simulink model "Frank_feedback"  (Simulink 8.3)
settings: Solver=ode4  StartTime=0.0  StopTime=30  FixedStep=Ts  RelTol=1e-3
values from neighbouring files (symbols this model uses):
  Ts = 0.001    [init_frank.m]
undefined symbols (not defined in the file or in its folder): K_lqr, Kt, R, rob_str, W
undefined symbols (not defined in the file): prjname
(part 1 of 2)
settings Model: Creator=parallels  LastModifiedBy=parallels
settings DataIOCC: SignalLoggingSaveFormat=Dataset
settings DebuggingCC: UnderspecifiedInitializationDetection=Simplified  StateNameClashWarn=none
settings GRTTargetCC: CombineOutputUpdateFcns=on  GRTInterface=off

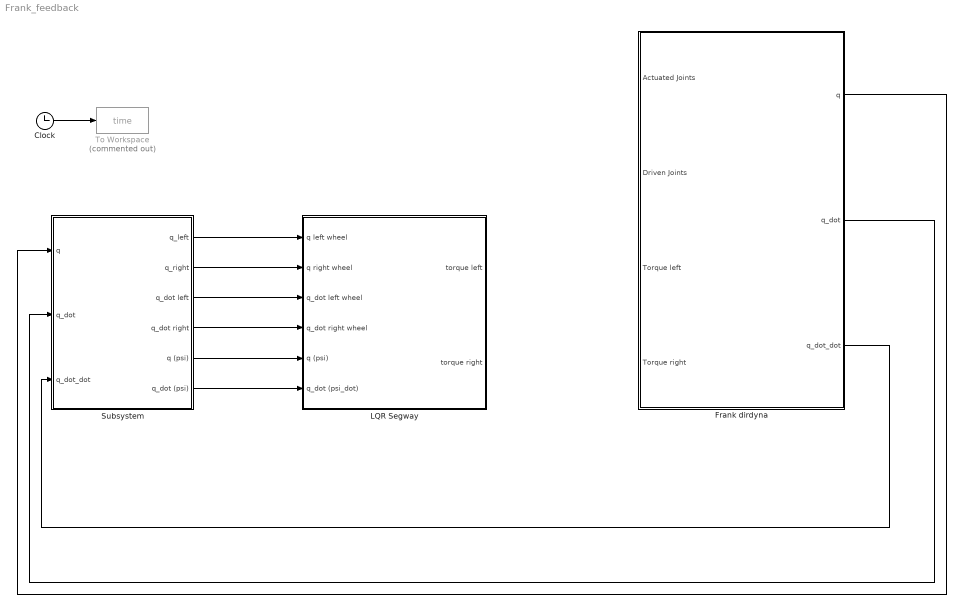
== system Frank_feedback ==
  Clock : Clock
  Frank dirdyna : Subsystem
  LQR Segway : Subsystem
  Subsystem : Subsystem
  To Workspace : ToWorkspace  Commented=on  VariableName=time  SampleTime=-1
  wires:
  Subsystem/1(q_left) -> LQR Segway/1("q left wheel ")
  Subsystem/2(q_right) -> LQR Segway/2(q right wheel)
  Subsystem/3(q_dot left) -> LQR Segway/3(q_dot left wheel)
  Subsystem/4(q_dot right) -> LQR Segway/4(q_dot right wheel)
  Subsystem/5(q (psi)) -> LQR Segway/5(q (psi))
  Subsystem/6(q_dot (psi)) -> LQR Segway/6("q_dot (psi_dot) ")
  Frank dirdyna/3(q_dot_dot) -> Subsystem/3(q_dot_dot)
  Frank dirdyna/2(q_dot) -> Subsystem/2(q_dot)
  Frank dirdyna/1(q) -> Subsystem/1(q)
  Clock/1 -> To Workspace/1

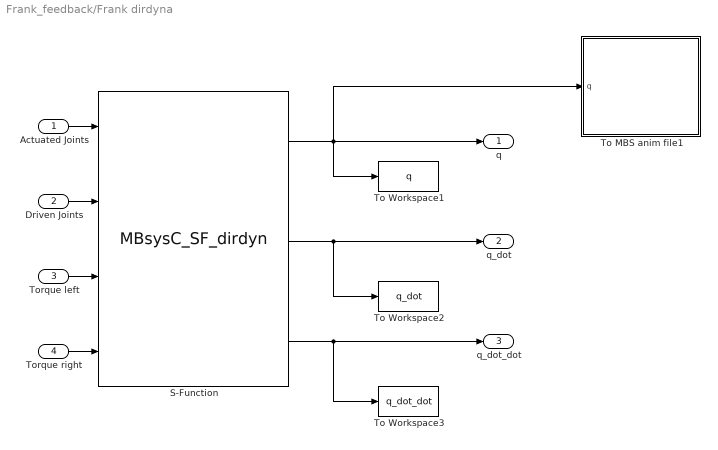
== system Frank_feedback/Frank dirdyna ==
  Actuated Joints : Inport
  Driven Joints : Inport  Port=2
  Torque left : Inport  Port=3
  Torque right : Inport  Port=4
  S-Function : S-Function  FunctionName=MBsysC_SF_dirdyn  Parameters='/home/parallels/Documents/MBProjects/Frank_segway/dataR/Frank_segway.mbs'  EnableBusSupport=off
  To MBS anim file1 : Subsystem  AncestorBlock=Robotran/Utilities/To MBS anim file  StopFcn=|  mask{varname=tqres, filename=simdir.anim, overwrite=0, samplingRate=1000, prjname=prjname}
      | varname = get_param(gcb,'varname');                                     
      | filename = get_param(gcb,'filename');                                   
      | tq = evalin('base',varname);                                            
      | tt = tq.time;                                                           
      | qq = tq.signals.values;                                                 
      | userData = get_param(gcb,'UserData');                                   
      | mbs_data = MBS_data;                                           
      | mbs_info = MBS_info;                                           
      | overwrite = str2double(get_param(gcb,'overwrite'));                     
      |                                                                         
      | samplingRate = str2double(get_param(gcb,'samplingRate'));               
      | mbs_gen_simdir(prjname,tt,qq,filename,overwrite,samplingRate);
      mask prompts: varname "variable name"; filename "anim file name"; overwrite "overwrite flag"; samplingRate "sampling rate"
      settings: CopyFcn=MBStoAnimFile_v2;  OpenFcn=MBStoAnimFile_v2;
      mask Display: image(imread('Logo_anim.jpg'))
  To Workspace1 : ToWorkspace  VariableName=q  SampleTime=-1
  To Workspace2 : ToWorkspace  VariableName=q_dot  SampleTime=-1
  To Workspace3 : ToWorkspace  VariableName=q_dot_dot  SampleTime=-1
  q : Outport
  q_dot : Outport  Port=2
  q_dot_dot : Outport  Port=3
  wires:
  Actuated Joints/1 -> S-Function/1
  Driven Joints/1 -> S-Function/2
  Torque left/1 -> S-Function/3
  Torque right/1 -> S-Function/4
  S-Function/1 -> To MBS anim file1/1(q), q/1, To Workspace1/1
  S-Function/2 -> To Workspace2/1, q_dot/1
  S-Function/3 -> q_dot_dot/1, To Workspace3/1

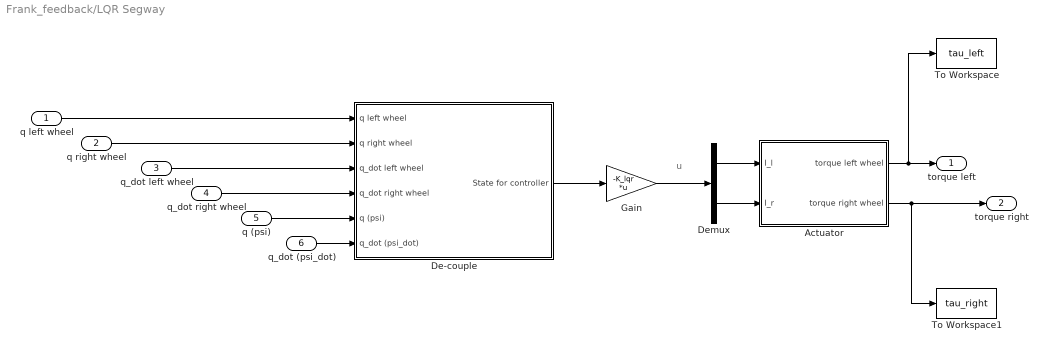
== system Frank_feedback/LQR Segway ==
  note: u
  "q left wheel " : Inport
  q right wheel : Inport  Port=2
  q_dot left wheel : Inport  Port=3
  q_dot right wheel : Inport  Port=4
  q (psi) : Inport  Port=5
  "q_dot (psi_dot) " : Inport  Port=6
  Actuator : Subsystem
  De-couple : Subsystem
  Demux : Demux  Outputs=2
  Gain : Gain  Gain=-K_lqr  Multiplication=Matrix(K*u) (u vector)
  To Workspace : ToWorkspace  VariableName=tau_left  SampleTime=-1
  To Workspace1 : ToWorkspace  VariableName=tau_right  SampleTime=-1
  torque left : Outport
  torque right : Outport  Port=2
  wires:
  "q left wheel "/1 -> De-couple/1("q left wheel ")
  q right wheel/1 -> De-couple/2(q right wheel)
  q_dot left wheel/1 -> De-couple/3(q_dot left wheel)
  q_dot right wheel/1 -> De-couple/4(q_dot right wheel)
  De-couple/1(State for controller) -> Gain/1
  q (psi)/1 -> De-couple/5(q (psi))
  "q_dot (psi_dot) "/1 -> De-couple/6("q_dot (psi_dot) ")
  Gain/1 -> Demux/1
  Actuator/1(torque left wheel) -> To Workspace/1, torque left/1
  Demux/1 -> Actuator/1(I_l)
  Demux/2 -> Actuator/2(I_r)
  Actuator/2(torque right wheel) -> To Workspace1/1, torque right/1

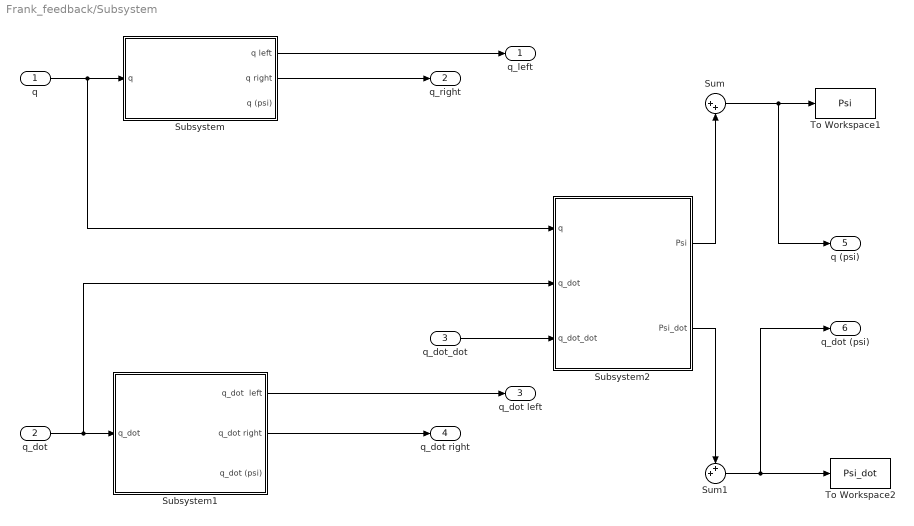
== system Frank_feedback/Subsystem ==
  q : Inport
  q_dot : Inport  Port=2
  q_dot_dot : Inport  Port=3
  Subsystem : Subsystem
  Subsystem1 : Subsystem
  Subsystem2 : Subsystem
  Sum : Sum  Inputs=|++
  Sum1 : Sum  Inputs=++|
  To Workspace1 : ToWorkspace  VariableName=Psi  SampleTime=-1
  To Workspace2 : ToWorkspace  VariableName=Psi_dot  SampleTime=-1
  q_left : Outport
  q_right : Outport  Port=2
  q_dot left : Outport  Port=3
  q_dot right : Outport  Port=4
  q (psi) : Outport  Port=5
  q_dot (psi) : Outport  Port=6
  wires:
  q/1 -> Subsystem2/1(q), Subsystem/1(q)
  Subsystem/2(q right) -> q_right/1
  Subsystem/1(q left) -> q_left/1
  q_dot/1 -> Subsystem2/2(q_dot), Subsystem1/1(q_dot)
  Subsystem1/2(q_dot right) -> q_dot right/1
  Subsystem1/1(q_dot  left) -> q_dot left/1
  q_dot_dot/1 -> Subsystem2/3(q_dot_dot)
  Sum1/1 -> q_dot (psi)/1, To Workspace2/1
  Sum/1 -> q (psi)/1, To Workspace1/1
  Subsystem2/1(Psi) -> Sum/2
  Subsystem2/2(Psi_dot) -> Sum1/1

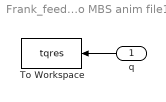
== system Frank_feedback/Frank dirdyna/To MBS anim file1 ==
  q : Inport
  To Workspace : ToWorkspace  VariableName=tqres  SaveFormat=Structure With Time  SampleTime=-1
  wires:
  q/1 -> To Workspace/1

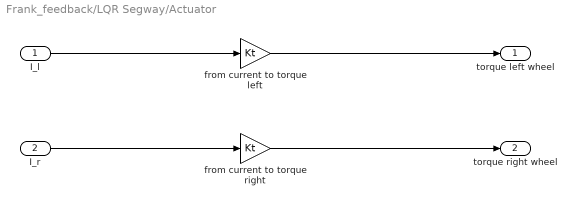
== system Frank_feedback/LQR Segway/Actuator ==
  I_l : Inport
  I_r : Inport  Port=2
  from current to torque left : Gain  Gain=Kt
  from current to torque right : Gain  Gain=Kt
  torque left wheel : Outport
  torque right wheel : Outport  Port=2
  wires:
  I_l/1 -> from current to torque left/1
  I_r/1 -> from current to torque right/1
  from current to torque left/1 -> torque left wheel/1
  from current to torque right/1 -> torque right wheel/1

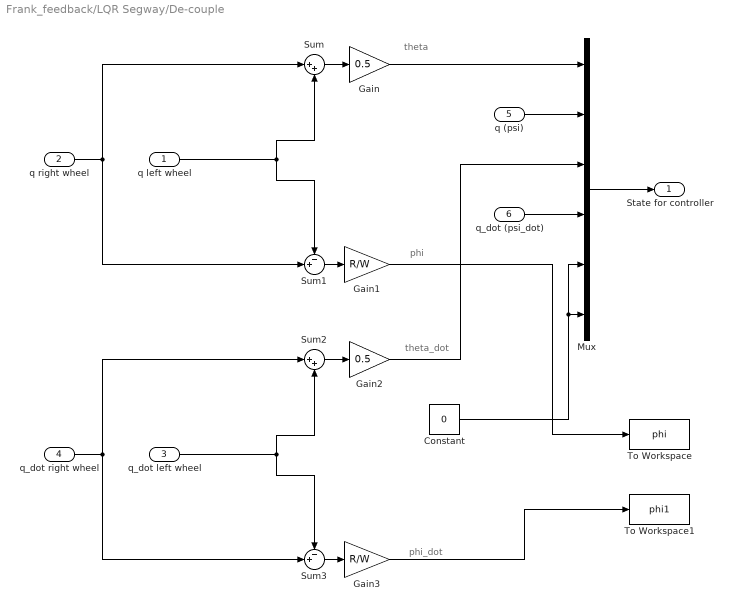
== system Frank_feedback/LQR Segway/De-couple ==
  note: phi
  note: theta
  note: phi_dot
  note: theta_dot
  "q left wheel " : Inport
  q right wheel : Inport  Port=2
  q_dot left wheel : Inport  Port=3
  q_dot right wheel : Inport  Port=4
  q (psi) : Inport  Port=5
  "q_dot (psi_dot) " : Inport  Port=6
  Constant : Constant  Value=0
  Gain : Gain  Gain=0.5
  Gain1 : Gain  Gain=R/W
  Gain2 : Gain  Gain=0.5
  Gain3 : Gain  Gain=R/W
  Mux : Mux  Inputs=6
  Sum : Sum  Inputs=|++
  Sum1 : Sum  Inputs=-+|
  Sum2 : Sum  Inputs=|++
  Sum3 : Sum  Inputs=-+|
  To Workspace : ToWorkspace  VariableName=phi  SampleTime=-1
  To Workspace1 : ToWorkspace  VariableName=phi1  SampleTime=-1
  State for controller : Outport
  wires:
  Sum1/1 -> Gain1/1
  q right wheel/1 -> Sum1/2, Sum/1
  Sum/1 -> Gain/1
  Sum3/1 -> Gain3/1
  Sum2/1 -> Gain2/1
  q_dot left wheel/1 -> Sum2/2, Sum3/1
  q_dot right wheel/1 -> Sum3/2, Sum2/1
  "q left wheel "/1 -> Sum/2, Sum1/1
  Gain/1 -> Mux/1
  q (psi)/1 -> Mux/2
  Gain2/1 -> Mux/3
  "q_dot (psi_dot) "/1 -> Mux/4
  Gain3/1 -> To Workspace1/1
  Mux/1 -> State for controller/1
  Gain1/1 -> To Workspace/1
  Constant/1 -> Mux/6, Mux/5

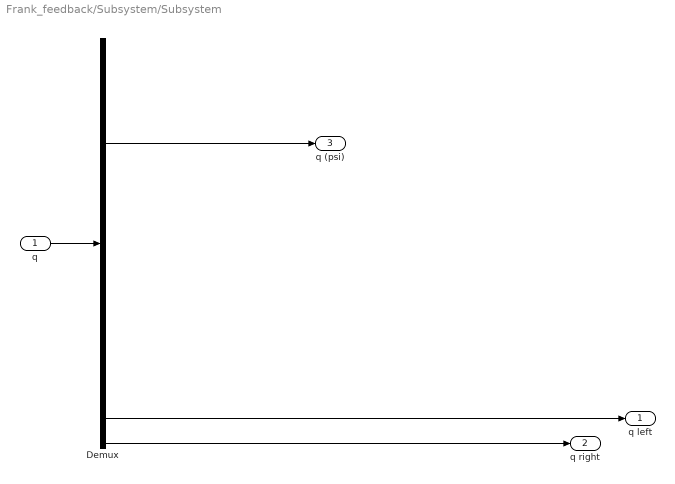
== system Frank_feedback/Subsystem/Subsystem ==
  q : Inport
  Demux : Demux  Outputs=17
  q left : Outport
  q right : Outport  Port=2
  q (psi) : Outport  Port=3
  wires:
  q/1 -> Demux/1
  Demux/17 -> q right/1
  Demux/16 -> q left/1
  Demux/5 -> q (psi)/1

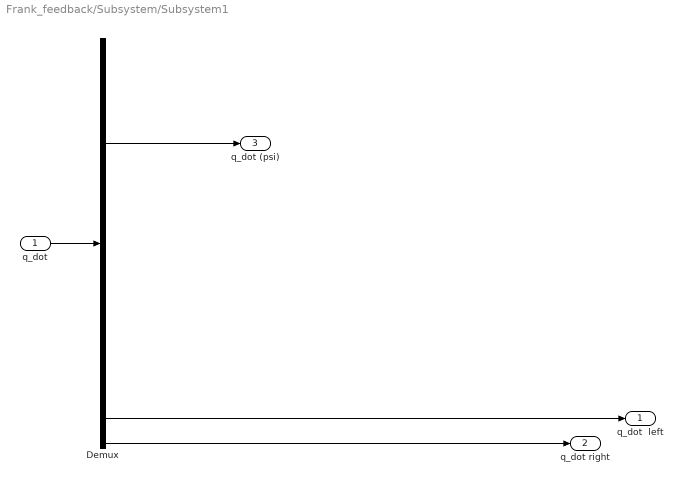
== system Frank_feedback/Subsystem/Subsystem1 ==
  q_dot : Inport
  Demux : Demux  Outputs=17
  q_dot  left : Outport
  q_dot right : Outport  Port=2
  q_dot (psi) : Outport  Port=3
  wires:
  q_dot/1 -> Demux/1
  Demux/17 -> q_dot right/1
  Demux/16 -> q_dot  left/1
  Demux/5 -> q_dot (psi)/1

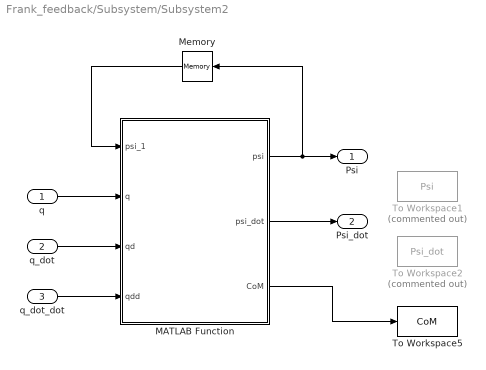
== system Frank_feedback/Subsystem/Subsystem2 ==
  q : Inport
  q_dot : Inport  Port=2
  q_dot_dot : Inport  Port=3
  MATLAB Function : MATLAB Function  TreatAsAtomicUnit=on
  Memory : Memory  InheritSampleTime=on
  To Workspace1 : ToWorkspace  Commented=on  VariableName=Psi  SampleTime=-1
  To Workspace2 : ToWorkspace  Commented=on  VariableName=Psi_dot  SampleTime=-1
  To Workspace5 : ToWorkspace  VariableName=CoM  SampleTime=-1
  Psi : Outport
  Psi_dot : Outport  Port=2
  wires:
  q/1 -> MATLAB Function/2(q)
  q_dot/1 -> MATLAB Function/3(qd)
  q_dot_dot/1 -> MATLAB Function/4(qdd)
  MATLAB Function/3(CoM) -> To Workspace5/1
  MATLAB Function/2(psi_dot) -> Psi_dot/1
  MATLAB Function/1(psi) -> Memory/1, Psi/1
  Memory/1 -> MATLAB Function/1(psi_1)
